simulink library "air_resistance"  (R2020b)
settings: Solver=VariableStepAuto  StartTime=0.0  StopTime=10.0  RelTol=1e-3
values from neighbouring files (symbols this model uses):
  Aproj = 2.5    [Projektskript.m]    (also in init.m)
  cw = 0.4    [Projektskript.m]    (also in init.m)
  rho = 1.2    [Projektskript.m]    (also in init.m)
settings Model: Creator=janbantle  LastModifiedBy=Johnathy

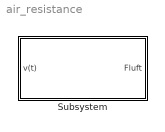
== system air_resistance ==
  Subsystem : Subsystem

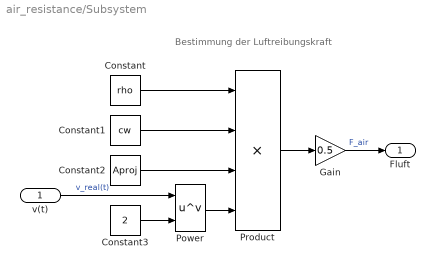
== system air_resistance/Subsystem ==
  note: Bestimmung der Luftreibungskraft
  v(t) : Inport
  Constant : Constant  Value=rho
  Constant1 : Constant  Value=cw
  Constant2 : Constant  Value=Aproj
  Constant3 : Constant  Value=2
  Gain : Gain  Gain=0.5
  Power : Math  Operator=pow  SaturateOnIntegerOverflow=on
  Product : Product  Inputs=4
  Fluft : Outport
  wires:
  Power/1 -> Product/4
  Constant3/1 -> Power/2
  Constant1/1 -> Product/2
  Product/1 -> Gain/1
  Gain/1 -> Fluft/1  "F_air"
  v(t)/1 -> Power/1  "v_real(t)"
  Constant2/1 -> Product/3
  Constant/1 -> Product/1
